simulink model "simple_PIL_model"  (Simulink 7.3)
settings: Solver=ode45  StartTime=0.0  StopTime=0.055  RelTol=1e-3
InitFcn:
  | % Processor selection for I/O assignment
  | % The chosen Target in the Coder Options window must match the selected MCU.
  | % Set the variable 'type_evm' to the following strings to choose a specific target:
  | 
  |   type_evm = 'TI28069';    % TI28069 Piccolo Launchpad
  | % type_evm = 'TI28377S';   % TI28377S Delfino Launchpad
  | % type_evm = 'TI28379LP';  % TI28379D Delfino Launchpad
  | % type_evm = 'TI280049C';  % TI280049C Piccolo Launchpad
  | % type_evm = 'TI28379CC';  % TI28379D Delfino Controlcard
  | % type_evm = 'TI28388D';   % TI28388D Controlcard
  | 
  | % Configure I/O based on processor
  | switch (type_evm)
  | 	case 'TI28069'
  | 	% Configuration for TI28069 Launchpad
  | 	%on the controller side	(compatible with BOOSTXL-DRV8305EVM)
  | 		ADC_DSP_IsenAB_Vdc = [3, 3+8, 5+8];
  | 		PWM_DSP_PWM = [4 5];
  | 		DO_DSP_LED = 34;
  | 		DI_DSP_En = 13;
  | 		PWR_DSP_Power = 27;
  | 		SCI_DSP = [28, 29];
  | 
  | 	case 'TI28377S'
  | 	% Configuration for TI28377S Launchpad
  | 	%on the controller side
  | 		ADC_DSP_IsenAB_Vdc = [4, 5, 3];
  | 		PWM_DSP_PWM = [8 9];
  | 		DO_DSP_LED = 12;
  | 		DI_DSP_En = 72;
  | 		PWR_DSP_Power = 43;
  | 		SCI_DSP = [85, 84];
  | 
  | 	case 'TI28379LP'
  | 	% Configuration for TI28379D Launchpad
  | 	%on the controller side
  | 		ADC_DSP_IsenAB_Vdc = [4, 3, 1];
  | 		PWM_DSP_PWM = [1 2];
  | 		DO_DSP_LED = 34;
  | 		DI_DSP_En = 124;
  | 		PWR_DSP_Power = 66;
  | 		SCI_DSP = [43, 42];
  | 
  | 	case 'TI280049C'
  | 	% Configuration for TI280049C Launchpad
  | 	%on the controller side
  | 		ADC_DSP_IsenAB_Vdc = [3, 6, 0];
  | 		PWM_DSP_PWM = [6 5];
  | 		DO_DSP_LED = 34;
  | 		DI_DSP_En = 58;
  | 		PWR_DSP_Power = 56;
  | 		SCI_DSP = [28, 29];
  | 
  | 		case 'TI28379CC'
  | 	% Configuration for TI28379D Controlcard
  | 	%on the controller side
  | 		ADC_DSP_IsenAB_Vdc = [1,2,3];
  | 		PWM_DSP_PWM = [1,2];
  | 		DO_DSP_LED = 34;
  | 		DI_DSP_En = 40;
  | 		PWR_DSP_Power = 39;
  | 		SCI_DSP = [28, 29];
  | 
  | 	case 'TI28388D'
  | 	% Configuration for TI28388D Controlcard
  | 	%on the controller side
  | 		ADC_DSP_IsenAB_Vdc = [1,2,3];
  | 		PWM_DSP_PWM = [1,2];
  | 		DO_DSP_LED = 34;
  | 		DI_DSP_En = 40;
  | 		PWR_DSP_Power = 39;
  | 		SCI_DSP = [28, 29];
  | 
  | 	otherwise
  | 	error('Unknown evaluation module selection, please choose either ''TI28069'', ''TI28377S'', ''TI28379LP'', ''TI280049C'', ''TI28379CC'' or ''TI28388D''.')
  | end
  | 
  | 
  | % switching frequency
  | fsw = 10e3; % switching frequency in Hz
  | 
  | % controller dicretizaton
  | Ts_controller = 1/fsw; % sample step size of the controller subsystem in sec
  | 
  | % current set point
  | ftoggle = fsw/200; % ~50 Hz
  | Iset_max= 3;     % current reference in A
  | Iset_min= -3;    % current reference in A
  | 
  | % input voltage
  | Vdc = 24; %input voltage in V
  | 
  | % test load
  | R = 1;      % load resistance in ohms
  | L = 250e-6; % load inductance in H
  | 
  | % PI current regulator design parameters
  | T_calc = 0.5*Ts_controller; % small time constant for control calculation
  | T_pwm = 0.5*Ts_controller; % small time constant for PWM output generation
  | T_sh = 0.5*Ts_controller; % small time constant for continuous time domain to digital conversion
  | T_delay = T_calc+T_pwm+T_sh; %one equivalent small time constant
  | 
  | K1 = 1/R;
  | Tn = L/R;
  | Ti = 2*K1*T_delay;
  | Kp = Tn/Ti;
  | Ki = 1/Ti;
  | 
  | %BOOSTXL-DRV8305EVM sensing gains
  | % voltage sensing gain (pole at 344.618 Hz)
  | Vm.R1 = 62000;
  | Vm.R2 = 4990;
  | Vm.C = 100e-9;
  | Vm.K = Vm.R2/(Vm.R1+Vm.R2);
  | Vm.T = Vm.C*Vm.R1*Vm.R2/(Vm.R1+Vm.R2)
  | 
  | % current sensing gain and offset
  | Im.K = 0.007*10;
  | Im.O = 3.3/2.0;
undefined symbols (not defined in the file): plecs
settings Model: Creator=kris  LastModifiedBy=manaswini  ExtModeTrigMode=oneshot  ExtModeArmWhenConnect=off  ExtModeAutoUpdateStatusClock=off
settings DataIOCC: LimitDataPoints=off  ReturnWorkspaceOutputs=off  SignalLoggingName=sigsOut
settings OptimizationCC: BooleanDataType=off  ExpressionDepthLimit=128  InitFltsAndDblsToZero=on
settings DebuggingCC: SaveWithParameterizedLinksMsg=none  SignalResolutionControl=TryResolveAllWithWarning  SolverPrmCheckMsg=none  MultiTaskDSMMsg=warning  MultiTaskCondExecSysMsg=none  FcnCallInpInsideContextMsg=Enable All  StrictBusMsg=ErrorLevel1
settings HardwareCC: TargetHWDeviceType=32-bit Generic  TargetUnknown=on  ProdEqTarget=off
settings RTWCC: IncludeERTFirstTime=on
settings CodeAppCC: CustomSymbolStrType=$N$R$M_T
settings GRTTargetCC: TargetFcnLib=ansi_tfl_tmw.mat  TargetFunctionLibrary=C89/C90 (ANSI)  ModelReferenceCompliant=off

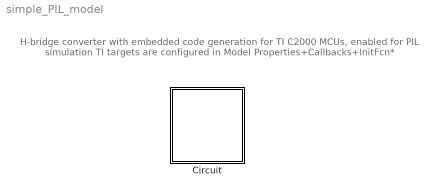
== system simple_PIL_model ==
  note: H-bridge converter
      | with embedded code generation for TI C2000 MCUs,
      | enabled for PIL simulation
      | TI targets are configured in Model Properties+Callbacks+InitFcn*
  Circuit : Subsystem  LoadFcn=plecs('sl', 200);  InitFcn=plecs('sl', 214);  StartFcn=plecs('sl', 208);  StopFcn=plecs('sl', 209);  ClipboardFcn=plecs('sl', 212, 22);  mask(PlecsCircuit){PLECSData=<binary blob, 15012 chars, not shown>}
      mask prompts: PLECSData "PLECS Data (Do not delete or modify!)"
      mask help: Drag this block into a Simulink model to create a new electrical circuit.
      mask init:
      | % PLACE CUSTOM INITIALIZATIONS ABOVE
      | % DO NOT REMOVE
      | plecs('sl', 215);
      | % DO NOT REMOVE
      settings: CopyFcn=plecs('sl', 203);  DeleteFcn=plecs('sl', 205);  UndoDeleteFcn=plecs('sl', 206);  PreSaveFcn=plecs('sl', 211);  PostSaveFcn=plecs('sl', 201);  NameChangeFcn=plecs('sl', 210);  DestroyFcn=plecs('sl', 207);  PreCopyFcn=plecs('sl', 216);  OpenFcn=plecs('sl', 202);  ErrorFcn=plerrorfcn
      mask Display: disp('PLECS\nCircuit')

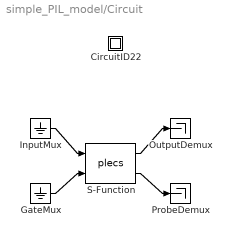
== system simple_PIL_model/Circuit ==
  " CircuitID22 " : Subsystem
  " GateMux " : Ground
  " InputMux " : Ground
  " OutputDemux " : Terminator
  " ProbeDemux " : Terminator
  " S-Function " : S-Function  FunctionName=plecs  EnableBusSupport=off
  wires:
  " InputMux "/1 -> " S-Function "/1
  " GateMux "/1 -> " S-Function "/2
  " S-Function "/1 -> " OutputDemux "/1
  " S-Function "/2 -> " ProbeDemux "/1

== system simple_PIL_model/Circuit/ CircuitID22  ==
